simulink model "Robot4_updated"  (R2022b)
settings: Solver=VariableStepAuto  StartTime=0.0  StopTime=300  FixedStep=0.001  RelTol=1e-3
values from neighbouring files (symbols this model uses):
  cn = 5    [parameters_Robot4_updated.m]
  ct = 1    [parameters_Robot4_updated.m]
  lambda = 0.0    (= 0)    [parameters_Robot4_updated.m]
undefined symbols (not defined in the file or in its folder): X, Y, Z
libraries: nesl_utility x57, sm_lib x39, slpidlib x6
(part 3 of 3)

== system Robot4_updated/Torque control 5 ==
  In1 : Inport
  PID Controller1 : slpidlib/PID Controller  Controller=PID  Form=Parallel  TimeDomain=Continuous-time  UseExternalTs=off  SampleTime=-1  IntegratorMethod=Forward Euler  FilterMethod=Forward Euler  ControllerParametersSource=internal  P=3  I=1  UseKiTs=off  D=0.05  N=1  UseFilter=on  TunerSelectOption=Transfer Function Based (PID Tuner App)  InitialConditionSource=internal  InitialConditionForIntegrator=0  InitialConditionForFilter=0  DifferentiatorICPrevScaledInput=0  ExternalReset=none  TrackingMode=off  Kt=1  LimitOutput=off  SatLimitsSource=internal  UpperSaturationLimit=inf  LowerSaturationLimit=-inf  LinearizeAsGain=on  AntiWindupMode=none  Kb=1  LimitIntegrator=off  UpperIntegratorSaturationLimit=inf  LowerIntegratorSaturationLimit=-inf  POutMin=[]  POutMax=[]  IOutMin=[]  IOutMax=[]  DOutMin=[]  DOutMax=[]  NOutMin=[]  NOutMax=[]  SumOutMin=[]  SumOutMax=[]  SaturationOutMin=[]  SaturationOutMax=[]  PParamMin=[]  PParamMax=[]  IParamMin=[]  IParamMax=[]  DParamMin=[]  DParamMax=[]  NParamMin=[]  NParamMax=[]  KbParamMin=[]  KbParamMax=[]  KtParamMin=[]  KtParamMax=[]  KbOutMin=[]  KbOutMax=[]  KtOutMin=[]  KtOutMax=[]  IntegratorOutMin=[]  IntegratorOutMax=[]  FilterOutMin=[]  FilterOutMax=[]  SumI1OutMin=[]  SumI1OutMax=[]  SumI2OutMin=[]  SumI2OutMax=[]  SumI3OutMin=[]  SumI3OutMax=[]  SumI4OutMin=[]  SumI4OutMax=[]  SumDOutMin=[]  SumDOutMax=[]  DifferentiatorOutMin=[]  DifferentiatorOutMax=[]  FilterDiffOutCoefMin=[]  FilterDiffOutCoefMax=[]  ReciprocalOutMin=[]  ReciprocalOutMax=[]  SumDenOutMin=[]  SumDenOutMax=[]  SumNumOutMin=[]  SumNumOutMax=[]  DivideOutMin=[]  DivideOutMax=[]  UdiffTsProdOutMin=[]  UdiffTsProdOutMax=[]  NTsProdOutMin=[]  NTsProdOutMax=[]  UintegralTsProdOutMin=[]  UintegralTsProdOutMax=[]  UngainTsProdOutMin=[]  UngainTsProdOutMax=[]  ClampingZeroOutDataTypeStr=Inherit: Inherit via back propagation  ClampingZeroOutMin=[]  ClampingZeroOutMax=[]  FilterDenConstantOutDataTypeStr=Inherit: Inherit via back propagation  FilterDenConstantOutMin=[]  FilterDenConstantOutMax=[]  PCopyOutDataTypeStr=Inherit: Inherit via back propagation  PCopyOutMin=[]  PCopyOutMax=[]  NCopyOutDataTypeStr=Inherit: Inherit via back propagation  NCopyOutMin=[]  NCopyOutMax=[]  IntegratorContinuousStateAttributes=''  IntegratorStateMustResolveToSignalObject=off  IntegratorRTWStateStorageClass=Auto  FilterContinuousStateAttributes=''  FilterStateMustResolveToSignalObject=off  FilterRTWStateStorageClass=Auto  ParallelPVariant=InternalParameters  IdealPVariant=Disabled  IVariant=InternalParameters  DVariant=InternalParameters  IntegratorVariant=Continuous  SatVariant=Disabled  AWVariant=Passthrough  PCopyVariant=Disabled  TRVariant=Disabled  FdbkBlocksVariant=Forward  IdealPFdbkVariant=Disabled  SatFdbkVariant=Disabled  DerivativeFilterVariant=ContFilter  NVariant=InternalParameters  NCopyVariant=Disabled  FilterICVariant=InternalICsFilter  IntegratorICVariant=InternalICs  ExternalResetVariant=Disabled  TRSumVariant=Passthrough  SumFdbkVariant=Disabled  SumVariant=Sum_PID  TsampFilterVariant=InternalTs  TsampNgainVariant=Passthrough  TsampIntegralVariant=Passthrough  ExternalSaturationOutDataTypeStr=Inherit: Same as second input
  PS-Simulink Converter2 : nesl_utility/PS-Simulink Converter  PhysicalDomain=network_engine_domain  SubClassName=ps_output  LeftPortType=input  RightPortType=output  PseudoPeriodic=off  Frequencies=[]  VectorFormat=1-D array  Unit=inherit  AffineConversion=off
  Simulink-PS Converter1 : nesl_utility/Simulink-PS Converter  PhysicalDomain=network_engine_domain  SubClassName=ps_input  LeftPortType=input  RightPortType=output  PseudoPeriodic=off  Frequencies=[]  NoiseDistribution=none  NoiseParameters=[]  Unit=N*m  AffineConversion=off  FilteringAndDerivatives=filter  SimscapeFilterOrder=2  InputFilterTimeConstant=0.001  UdotUserProvided=1
  Sum3 : Sum  Inputs=|+-
  output : PMIOPort  Side=Right
  input : PMIOPort  Port=2  Side=Left
  wires:
  PS-Simulink Converter2/1 -> Sum3/2
  Sum3/1 -> PID Controller1/1
  In1/1 -> Sum3/1
  PID Controller1/1 -> Simulink-PS Converter1/1
  connections:
  output/RConn1 -- Simulink-PS Converter1/RConn1
  PS-Simulink Converter2/LConn1 -- input/RConn1

== system Robot4_updated/Torque control 6 ==
  In1 : Inport
  PID Controller1 : slpidlib/PID Controller  Controller=PID  Form=Parallel  TimeDomain=Continuous-time  UseExternalTs=off  SampleTime=-1  IntegratorMethod=Forward Euler  FilterMethod=Forward Euler  ControllerParametersSource=internal  P=3  I=1  UseKiTs=off  D=0.05  N=1  UseFilter=on  TunerSelectOption=Transfer Function Based (PID Tuner App)  InitialConditionSource=internal  InitialConditionForIntegrator=0  InitialConditionForFilter=0  DifferentiatorICPrevScaledInput=0  ExternalReset=none  TrackingMode=off  Kt=1  LimitOutput=off  SatLimitsSource=internal  UpperSaturationLimit=inf  LowerSaturationLimit=-inf  LinearizeAsGain=on  AntiWindupMode=none  Kb=1  LimitIntegrator=off  UpperIntegratorSaturationLimit=inf  LowerIntegratorSaturationLimit=-inf  POutMin=[]  POutMax=[]  IOutMin=[]  IOutMax=[]  DOutMin=[]  DOutMax=[]  NOutMin=[]  NOutMax=[]  SumOutMin=[]  SumOutMax=[]  SaturationOutMin=[]  SaturationOutMax=[]  PParamMin=[]  PParamMax=[]  IParamMin=[]  IParamMax=[]  DParamMin=[]  DParamMax=[]  NParamMin=[]  NParamMax=[]  KbParamMin=[]  KbParamMax=[]  KtParamMin=[]  KtParamMax=[]  KbOutMin=[]  KbOutMax=[]  KtOutMin=[]  KtOutMax=[]  IntegratorOutMin=[]  IntegratorOutMax=[]  FilterOutMin=[]  FilterOutMax=[]  SumI1OutMin=[]  SumI1OutMax=[]  SumI2OutMin=[]  SumI2OutMax=[]  SumI3OutMin=[]  SumI3OutMax=[]  SumI4OutMin=[]  SumI4OutMax=[]  SumDOutMin=[]  SumDOutMax=[]  DifferentiatorOutMin=[]  DifferentiatorOutMax=[]  FilterDiffOutCoefMin=[]  FilterDiffOutCoefMax=[]  ReciprocalOutMin=[]  ReciprocalOutMax=[]  SumDenOutMin=[]  SumDenOutMax=[]  SumNumOutMin=[]  SumNumOutMax=[]  DivideOutMin=[]  DivideOutMax=[]  UdiffTsProdOutMin=[]  UdiffTsProdOutMax=[]  NTsProdOutMin=[]  NTsProdOutMax=[]  UintegralTsProdOutMin=[]  UintegralTsProdOutMax=[]  UngainTsProdOutMin=[]  UngainTsProdOutMax=[]  ClampingZeroOutDataTypeStr=Inherit: Inherit via back propagation  ClampingZeroOutMin=[]  ClampingZeroOutMax=[]  FilterDenConstantOutDataTypeStr=Inherit: Inherit via back propagation  FilterDenConstantOutMin=[]  FilterDenConstantOutMax=[]  PCopyOutDataTypeStr=Inherit: Inherit via back propagation  PCopyOutMin=[]  PCopyOutMax=[]  NCopyOutDataTypeStr=Inherit: Inherit via back propagation  NCopyOutMin=[]  NCopyOutMax=[]  IntegratorContinuousStateAttributes=''  IntegratorStateMustResolveToSignalObject=off  IntegratorRTWStateStorageClass=Auto  FilterContinuousStateAttributes=''  FilterStateMustResolveToSignalObject=off  FilterRTWStateStorageClass=Auto  ParallelPVariant=InternalParameters  IdealPVariant=Disabled  IVariant=InternalParameters  DVariant=InternalParameters  IntegratorVariant=Continuous  SatVariant=Disabled  AWVariant=Passthrough  PCopyVariant=Disabled  TRVariant=Disabled  FdbkBlocksVariant=Forward  IdealPFdbkVariant=Disabled  SatFdbkVariant=Disabled  DerivativeFilterVariant=ContFilter  NVariant=InternalParameters  NCopyVariant=Disabled  FilterICVariant=InternalICsFilter  IntegratorICVariant=InternalICs  ExternalResetVariant=Disabled  TRSumVariant=Passthrough  SumFdbkVariant=Disabled  SumVariant=Sum_PID  TsampFilterVariant=InternalTs  TsampNgainVariant=Passthrough  TsampIntegralVariant=Passthrough  ExternalSaturationOutDataTypeStr=Inherit: Same as second input
  PS-Simulink Converter2 : nesl_utility/PS-Simulink Converter  PhysicalDomain=network_engine_domain  SubClassName=ps_output  LeftPortType=input  RightPortType=output  PseudoPeriodic=off  Frequencies=[]  VectorFormat=1-D array  Unit=inherit  AffineConversion=off
  Simulink-PS Converter1 : nesl_utility/Simulink-PS Converter  PhysicalDomain=network_engine_domain  SubClassName=ps_input  LeftPortType=input  RightPortType=output  PseudoPeriodic=off  Frequencies=[]  NoiseDistribution=none  NoiseParameters=[]  Unit=N*m  AffineConversion=off  FilteringAndDerivatives=filter  SimscapeFilterOrder=2  InputFilterTimeConstant=0.001  UdotUserProvided=1
  Sum3 : Sum  Inputs=|+-
  output : PMIOPort  Side=Right
  input : PMIOPort  Port=2  Side=Left
  wires:
  PS-Simulink Converter2/1 -> Sum3/2
  Sum3/1 -> PID Controller1/1
  In1/1 -> Sum3/1
  PID Controller1/1 -> Simulink-PS Converter1/1
  connections:
  output/RConn1 -- Simulink-PS Converter1/RConn1
  PS-Simulink Converter2/LConn1 -- input/RConn1

== matlab function Robot4_updated/Link2/MATLAB Function ==
  data: vx input; fx output; vy input; ct input; cn input; th input; fy output
function [fx,fy] = fcn(vx,vy,ct,cn,th)
fx = -(ct*(cos(th))^2+cn*(sin(th))^2)*vx-((ct-cn)*sin(th)*cos(th))*vy;
fy = -((ct-cn)*sin(th)*cos(th))*vx-(ct*(sin(th))^2+cn*(cos(th))^2)*vy;
end

== matlab function Robot4_updated/Link1/MATLAB Function ==
  data: vx input; fx output; vy input; ct input; cn input; th input; fy output
function [fx,fy] = fcn(vx,vy,ct,cn,th)
fx = -(ct*(cos(th))^2+cn*(sin(th))^2)*vx-((ct-cn)*sin(th)*cos(th))*vy;
fy = -((ct-cn)*sin(th)*cos(th))*vx-(ct*(sin(th))^2+cn*(cos(th))^2)*vy;
end

== matlab function Robot4_updated/Link3/MATLAB Function ==
  data: vx input; fx output; vy input; ct input; cn input; th input; fy output
function [fx,fy] = fcn(vx,vy,ct,cn,th)
fx = -(ct*(cos(th))^2+cn*(sin(th))^2)*vx-((ct-cn)*sin(th)*cos(th))*vy;
fy = -((ct-cn)*sin(th)*cos(th))*vx-(ct*(sin(th))^2+cn*(cos(th))^2)*vy;
end

== matlab function Robot4_updated/Link4/MATLAB Function ==
  data: vx input; fx output; vy input; ct input; cn input; th input; fy output
function [fx,fy] = fcn(vx,vy,ct,cn,th)
fx = -(ct*(cos(th))^2+cn*(sin(th))^2)*vx-((ct-cn)*sin(th)*cos(th))*vy;
fy = -((ct-cn)*sin(th)*cos(th))*vx-(ct*(sin(th))^2+cn*(cos(th))^2)*vy;
end

== matlab function Robot4_updated/Link5/MATLAB Function ==
  data: vx input; fx output; vy input; ct input; cn input; th input; fy output
function [fx,fy] = fcn(vx,vy,ct,cn,th)
fx = -(ct*(cos(th))^2+cn*(sin(th))^2)*vx-((ct-cn)*sin(th)*cos(th))*vy;
fy = -((ct-cn)*sin(th)*cos(th))*vx-(ct*(sin(th))^2+cn*(cos(th))^2)*vy;
end

== matlab function Robot4_updated/Link6/MATLAB Function ==
  data: vx input; fx output; vy input; ct input; cn input; th input; fy output
function [fx,fy] = fcn(vx,vy,ct,cn,th)
fx = -(ct*(cos(th))^2+cn*(sin(th))^2)*vx-((ct-cn)*sin(th)*cos(th))*vy;
fy = -((ct-cn)*sin(th)*cos(th))*vx-(ct*(sin(th))^2+cn*(cos(th))^2)*vy;
end

== matlab function Robot4_updated/Link7/MATLAB Function ==
  data: vx input; fx output; vy input; ct input; cn input; th input; fy output
function [fx,fy] = fcn(vx,vy,ct,cn,th)
fx = -(ct*(cos(th))^2+cn*(sin(th))^2)*vx-((ct-cn)*sin(th)*cos(th))*vy;
fy = -((ct-cn)*sin(th)*cos(th))*vx-(ct*(sin(th))^2+cn*(cos(th))^2)*vy;
end
